simulink model "windup2"  (R2018a)
settings: Solver=VariableStepAuto  StartTime=0.0  StopTime=Tmax  RelTol=1e-3
values from neighbouring files (symbols this model uses):
  Kd = 2.7    [windup2_test.m]
  N = numel(Gall)    [ultgain.m]    (also in windup2_test.m = 10; windup_test.m = 10)
  S = 0.1    [windup2_test.m]    (also in windup_test.m = 4)
  Td = 0.8    [windup2_test.m]    (also in windup_test.m = 1)
  Ti = 7.5    [windup2_test.m]    (also in windup_test.m = 1; workshop7.m = 1.6)
  Tt = sqrt(Ti*Td)    [windup2_test.m]
settings Model: Creator=will  LastModifiedBy=will

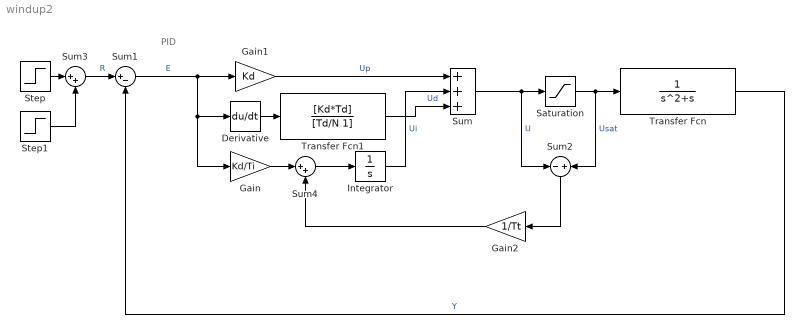
== system windup2 ==
  note: PID
  Derivative : Derivative
  Gain : Gain  Gain=Kd/Ti
  Gain1 : Gain  Gain=Kd
  Gain2 : Gain  Gain=1/Tt
  Integrator : Integrator
  Saturation : Saturate  UpperLimit=S  LowerLimit=-S
  Step : Step  SampleTime=0
  Step1 : Step  Time=100  After=-1  SampleTime=0
  Sum : Sum  Inputs=+++
  Sum1 : Sum  Inputs=|+-
  Sum2 : Sum  Inputs=-|+
  Sum3 : Sum  Inputs=|++
  Sum4 : Sum  Inputs=|++
  Transfer Fcn : TransferFcn  Denominator=[1 1 0]
  Transfer Fcn1 : TransferFcn  Numerator=[Kd*Td]  Denominator=[Td/N 1]
  wires:
  Gain1/1 -> Sum/1  "Up"
  Integrator/1 -> Sum/2  "Ui"
  Transfer Fcn1/1 -> Sum/3  "Ud"
  Sum1/1 -> Gain/1, Derivative/1, Gain1/1  "E"
  Sum/1 -> Sum2/1, Saturation/1  "U"
  Derivative/1 -> Transfer Fcn1/1
  Saturation/1 -> Sum2/2, Transfer Fcn/1  "Usat"
  Transfer Fcn/1 -> Sum1/2  "Y"
  Step1/1 -> Sum3/2
  Step/1 -> Sum3/1
  Sum3/1 -> Sum1/1  "R"
  Gain/1 -> Sum4/1
  Sum4/1 -> Integrator/1
  Sum2/1 -> Gain2/1
  Gain2/1 -> Sum4/2
